simulink model "detectors"  (R2019b)
settings: Solver=VariableStepAuto  StartTime=0.0  StopTime=10.0  RelTol=1e-3
values from neighbouring files (symbols this model uses):
  beta = 0.01    [var.mat]
  c = 2    [var.mat]
  m = 4    [var.mat]
  mu = 0.8    [var.mat]
  omega = 1    [var.mat]
  r = 5    [var.mat]
  s = 1.5    [var.mat]
  steadyVal = 10    [var.mat]
  zeta = 0.5    [var.mat]
libraries: mySTLLib x28
settings Model: Creator=yuxia  LastModifiedBy=yuxia
settings SolverCC: ZeroCrossAlgorithm=Adaptive
settings DebuggingCC: IgnoredZcDiagnostic=none

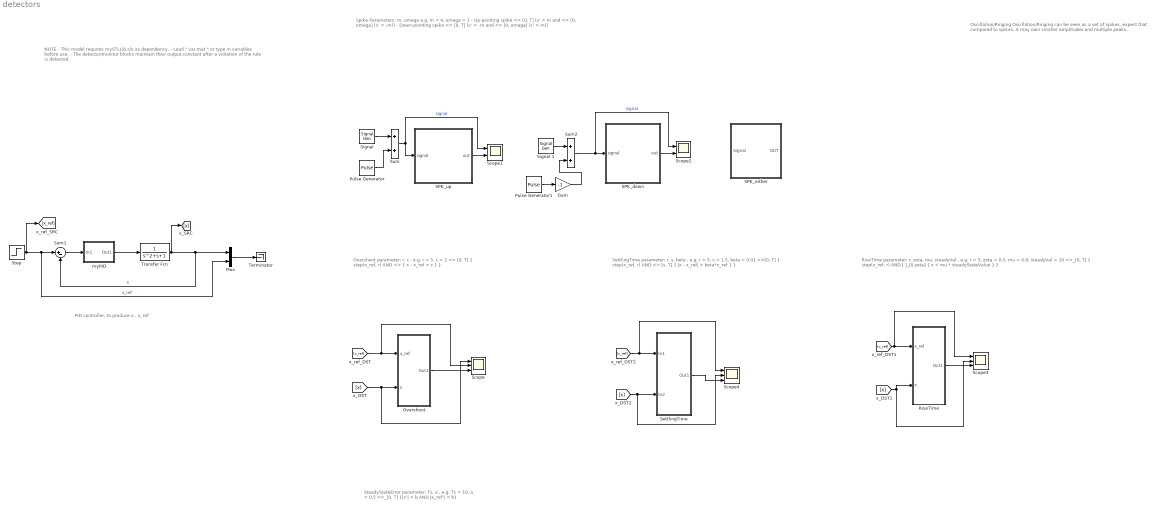
== system detectors ==
  note: PID controller, to produce x , x_ref
  note: Overshoot
      |
      | parameter: r, c , e.g. r = 5, c = 2
      | <> [0, T] { step(x_ref, r) AND <> { x - x_ref > c } }
  note: NOTE
      |
      | - This model requires mySTLLib.slx as dependency.
      |
      | - Load " var.mat " or type in variables before use.
      |
      | - The detector/monitor blocks maintain their output constant after a violation of the rule is detected.
  note: Spike
      |
      | Parameters: m, omega e.g. m = 4, omega = 1
      |
      | - Up-pointing spike
      | <> [0, T] (s' > m and <> [0, omega] (s' < -m))
      |
      | - Down-pointing spike
      | <> [0, T] (s' < -m and <> [0, omega] (s' > m))
  note: Oscillation/Ringing
      |
      | Oscillation/Ringing can be seen as a set of spikes, expect that compared to spikes, it may own smaller amplitudes and multiple peaks.
  note: SettlingTime
      |
      | parameter: r, s, beta , e.g. r = 5, s = 1.5, beta = 0.01
      |
      | <>[0, T] { step(x_ref, r) AND <> [s, T] { |x - x_ref| > beta*x_ref } }
  note: RiseTime
      |
      | parameter: r, zeta, mu, steadyVal , e.g. r = 5, zeta = 0.5, mu = 0.8, steadyVal = 10
      |
      | <>_[0, T] { step(x_ref, r) AND [ ]_[0,zeta] { x < mu * steadyStateValue } }
  note: SteadyStateError
      |
      | parameter: Ts, a , e.g. Ts = 10, a = 0.5
      |
      | <>_[0, T] {|x'| < b AND |x_ref'| < b}
  Gain : Gain  Gain=-1
  Mux : Mux  Inputs=2
  Overshoot : Subsystem
  Pulse Generator : DiscretePulseGenerator  PulseType=Time based  Period=10  PhaseDelay=3.3
  Pulse Generator1 : DiscretePulseGenerator  PulseType=Time based  Period=10  PhaseDelay=3.3
  RiseTime : Subsystem
  SPK_down : Subsystem
  SPK_either : Subsystem
  SPK_up : Subsystem
  Scope : Scope  NumInputPorts=3
  Scope1 : Scope  NumInputPorts=2
  Scope2 : Scope  NumInputPorts=2
  Scope3 : Scope  NumInputPorts=3
  Scope4 : Scope  NumInputPorts=3
  SettlingTime : Subsystem
  "Signal " : SignalGenerator  WaveForm=square  Units=rad/sec
  Signal 1 : SignalGenerator  WaveForm=square  Units=rad/sec
  Step : Step  After=10  SampleTime=0
  Sum : Sum
  Sum1 : Sum  Inputs=|+-
  Sum2 : Sum
  Terminator : Terminator
  Transfer Fcn : TransferFcn  Denominator=[1 1 1]
  myPID : Subsystem
  wires:
  SPK_up/1("out ") -> Scope1/2
  "Signal "/1 -> Sum/1
  Sum/1 -> Scope1/1, SPK_up/1(signal)  "signal"
  [x_ref] -> Scope/2, Overshoot/1(x_ref)
  [x] -> Scope/1, Overshoot/2(x)
  Overshoot/1(Out1) -> Scope/3
  Transfer Fcn/1 -> Mux/1, Sum1/2, [x]  "x"
  myPID/1(Out1) -> Transfer Fcn/1
  Step/1 -> Mux/2, Sum1/1, [x_ref]  "x_ref"
  Sum1/1 -> myPID/1(In1)
  Mux/1 -> Terminator/1
  Sum2/1 -> Scope2/1, SPK_down/1(signal)  "signal"
  SPK_down/1("out ") -> Scope2/2
  Pulse Generator1/1 -> Gain/1
  Signal 1/1 -> Sum2/1
  [x_ref] -> Scope4/1, SettlingTime/1(In1)
  [x] -> SettlingTime/2(In2), Scope4/2
  SettlingTime/1(Out1) -> Scope4/3
  Gain/1 -> Sum2/2
  Pulse Generator/1 -> Sum/2
  [x_ref] -> Scope3/1, RiseTime/1("x_ref ")
  [x] -> Scope3/2, RiseTime/2(x)
  RiseTime/1(Out1) -> Scope3/3

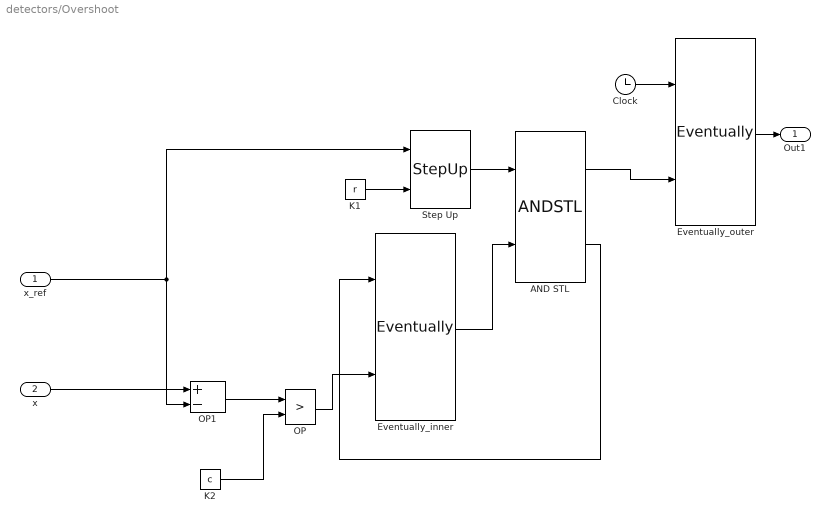
== system detectors/Overshoot ==
  x_ref : Inport
  x : Inport  Port=2
  AND STL : mySTLLib/ANDSTL  SystemSampleTime=-1  Latency=0  AutoFrameSizeCalculation=off
      settings: SourceProductName=My STL Library
  Clock : Clock
  Eventually_inner : mySTLLib/Eventually  SystemSampleTime=-1  Latency=0  AutoFrameSizeCalculation=off
      settings: SourceProductName=My STL Library
  Eventually_outer : mySTLLib/Eventually  SystemSampleTime=-1  Latency=0  AutoFrameSizeCalculation=off
      settings: SourceProductName=My STL Library
  "K1 " : Constant  Value=r
  K2 : Constant  Value=c
  OP : RelationalOperator  Operator=>  OutDataTypeStr=boolean  RndMeth=Simplest
  OP1 : Sum  Inputs=+-
  Step Up : mySTLLib/StepUp  SystemSampleTime=-1  Latency=0  AutoFrameSizeCalculation=off
      settings: SourceProductName=My STL Library
  Out1 : Outport
  wires:
  "K1 "/1 -> Step Up/2
  AND STL/2 -> Eventually_inner/1
  x/1 -> OP1/1
  OP1/1 -> OP/1
  Eventually_outer/1 -> Out1/1
  x_ref/1 -> Step Up/1, OP1/2
  Step Up/1 -> AND STL/1
  OP/1 -> Eventually_inner/2
  AND STL/1 -> Eventually_outer/2
  K2/1 -> OP/2
  Clock/1 -> Eventually_outer/1
  Eventually_inner/1 -> AND STL/2

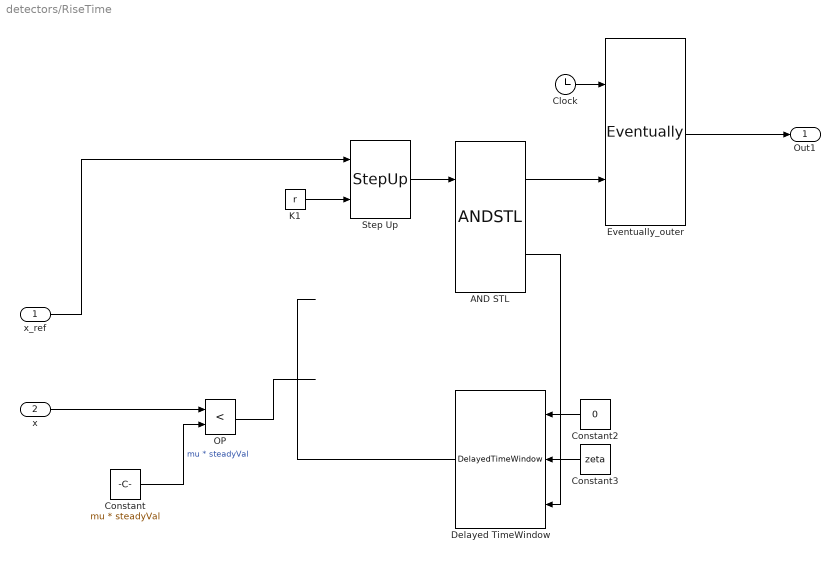
== system detectors/RiseTime ==
  "x_ref " : Inport
  x : Inport  Port=2
  AND STL : mySTLLib/ANDSTL  SystemSampleTime=-1  Latency=0  AutoFrameSizeCalculation=off
      settings: SourceProductName=My STL Library
  Clock : Clock
  Constant : Constant  Value=mu * steadyVal
  Constant2 : Constant  Value=0
  Constant3 : Constant  Value=zeta
  Delayed TimeWindow : mySTLLib/DelayedTimeWindow  SystemSampleTime=-1  Latency=0  AutoFrameSizeCalculation=off
      settings: SourceProductName=My STL Library
  Eventually_outer : mySTLLib/Eventually  SystemSampleTime=-1  Latency=0  AutoFrameSizeCalculation=off
      settings: SourceProductName=My STL Library
  "K1 " : Constant  Value=r
  OP : RelationalOperator  Operator=<  OutDataTypeStr=boolean  RndMeth=Simplest
  Step Up : mySTLLib/StepUp  SystemSampleTime=-1  Latency=0  AutoFrameSizeCalculation=off
      settings: SourceProductName=My STL Library
  Out1 : Outport
  wires:
  "K1 "/1 -> Step Up/2
  Constant/1 -> OP/2  "mu * steadyVal"
  AND STL/1 -> Eventually_outer/2
  Eventually_outer/1 -> Out1/1
  "x_ref "/1 -> Step Up/1
  ? -> AND STL/2
  Clock/1 -> Eventually_outer/1
  Step Up/1 -> AND STL/1
  Constant2/1 -> Delayed TimeWindow/1
  Constant3/1 -> Delayed TimeWindow/2
  AND STL/2 -> Delayed TimeWindow/3
  x/1 -> OP/1
  OP/1 -> ?
  Delayed TimeWindow/1 -> ?

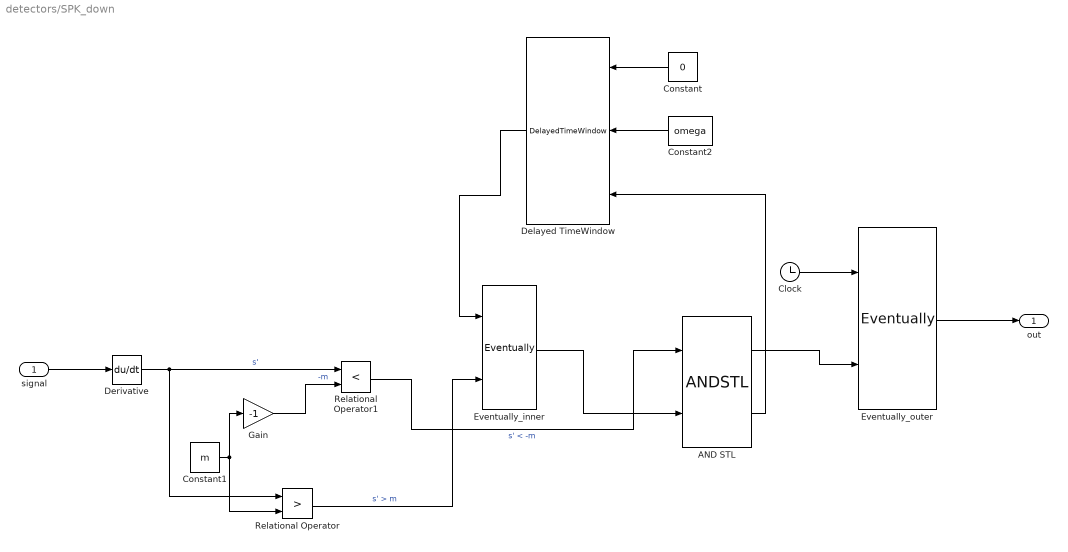
== system detectors/SPK_down ==
  signal : Inport
  AND STL : mySTLLib/ANDSTL  SystemSampleTime=-1  Latency=0  AutoFrameSizeCalculation=off
      settings: SourceProductName=My STL Library
  Clock : Clock
  Constant : Constant  Value=0
  Constant1 : Constant  Value=m
  Constant2 : Constant  Value=omega
  Delayed TimeWindow : mySTLLib/DelayedTimeWindow  SystemSampleTime=-1  Latency=0  AutoFrameSizeCalculation=off
      settings: SourceProductName=My STL Library
  Derivative : Derivative
  Eventually_inner : mySTLLib/Eventually  SystemSampleTime=-1  Latency=0  AutoFrameSizeCalculation=off
      settings: SourceProductName=My STL Library
  Eventually_outer : mySTLLib/Eventually  SystemSampleTime=-1  Latency=0  AutoFrameSizeCalculation=off
      settings: SourceProductName=My STL Library
  Gain : Gain  Gain=-1
  Relational Operator : RelationalOperator  Operator=>  OutDataTypeStr=boolean  RndMeth=Simplest
  Relational Operator1 : RelationalOperator  Operator=<  OutDataTypeStr=boolean  RndMeth=Simplest
  "out " : Outport
  wires:
  Clock/1 -> Eventually_outer/1
  Constant2/1 -> Delayed TimeWindow/2
  Constant1/1 -> Gain/1, Relational Operator/2
  signal/1 -> Derivative/1
  AND STL/2 -> Delayed TimeWindow/3
  Delayed TimeWindow/1 -> Eventually_inner/1
  Eventually_outer/1 -> "out "/1
  Derivative/1 -> Relational Operator1/1, Relational Operator/1  "s'"
  Relational Operator/1 -> Eventually_inner/2  "s' > m"
  Eventually_inner/1 -> AND STL/2
  Constant/1 -> Delayed TimeWindow/1
  Gain/1 -> Relational Operator1/2  "-m"
  AND STL/1 -> Eventually_outer/2
  Relational Operator1/1 -> AND STL/1  "s' < -m"

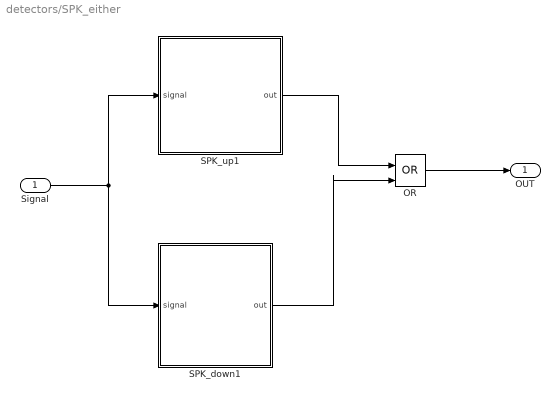
== system detectors/SPK_either ==
  Signal : Inport
  OR : Logic  Operator=OR  IconShape=distinctive  AllPortsSameDT=off  OutDataTypeStr=boolean
  SPK_down1 : Subsystem
  SPK_up1 : Subsystem
  OUT : Outport
  wires:
  Signal/1 -> SPK_up1/1(signal), SPK_down1/1(signal)
  OR/1 -> OUT/1
  SPK_up1/1("out ") -> OR/1
  SPK_down1/1("out ") -> OR/2

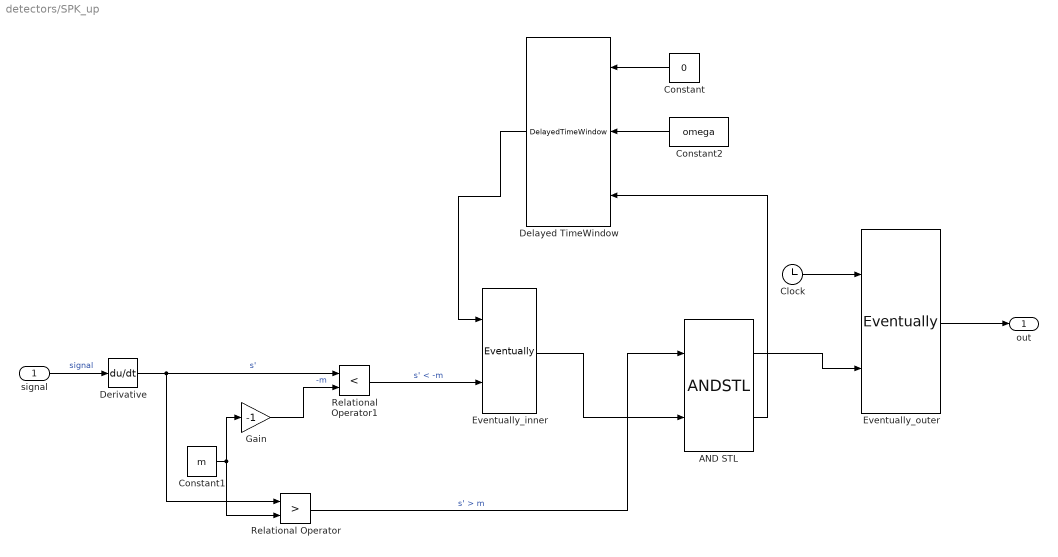
== system detectors/SPK_up ==
  signal : Inport
  AND STL : mySTLLib/ANDSTL  SystemSampleTime=-1  Latency=0  AutoFrameSizeCalculation=off
      settings: SourceProductName=My STL Library
  Clock : Clock
  Constant : Constant  Value=0
  Constant1 : Constant  Value=m
  Constant2 : Constant  Value=omega
  Delayed TimeWindow : mySTLLib/DelayedTimeWindow  SystemSampleTime=-1  Latency=0  AutoFrameSizeCalculation=off
      settings: SourceProductName=My STL Library
  Derivative : Derivative
  Eventually_inner : mySTLLib/Eventually  SystemSampleTime=-1  Latency=0  AutoFrameSizeCalculation=off
      settings: SourceProductName=My STL Library
  Eventually_outer : mySTLLib/Eventually  SystemSampleTime=-1  Latency=0  AutoFrameSizeCalculation=off
      settings: SourceProductName=My STL Library
  Gain : Gain  Gain=-1
  Relational Operator : RelationalOperator  Operator=>  OutDataTypeStr=boolean  RndMeth=Simplest
  Relational Operator1 : RelationalOperator  Operator=<  OutDataTypeStr=boolean  RndMeth=Simplest
  "out " : Outport
  wires:
  signal/1 -> Derivative/1  "signal"
  Eventually_outer/1 -> "out "/1
  Clock/1 -> Eventually_outer/1
  AND STL/1 -> Eventually_outer/2
  Gain/1 -> Relational Operator1/2  "-m"
  Derivative/1 -> Relational Operator1/1, Relational Operator/1  "s'"
  Relational Operator/1 -> AND STL/1  "s' > m"
  Constant1/1 -> Gain/1, Relational Operator/2
  Relational Operator1/1 -> Eventually_inner/2  "s' < -m"
  Eventually_inner/1 -> AND STL/2
  Delayed TimeWindow/1 -> Eventually_inner/1
  AND STL/2 -> Delayed TimeWindow/3
  Constant/1 -> Delayed TimeWindow/1
  Constant2/1 -> Delayed TimeWindow/2

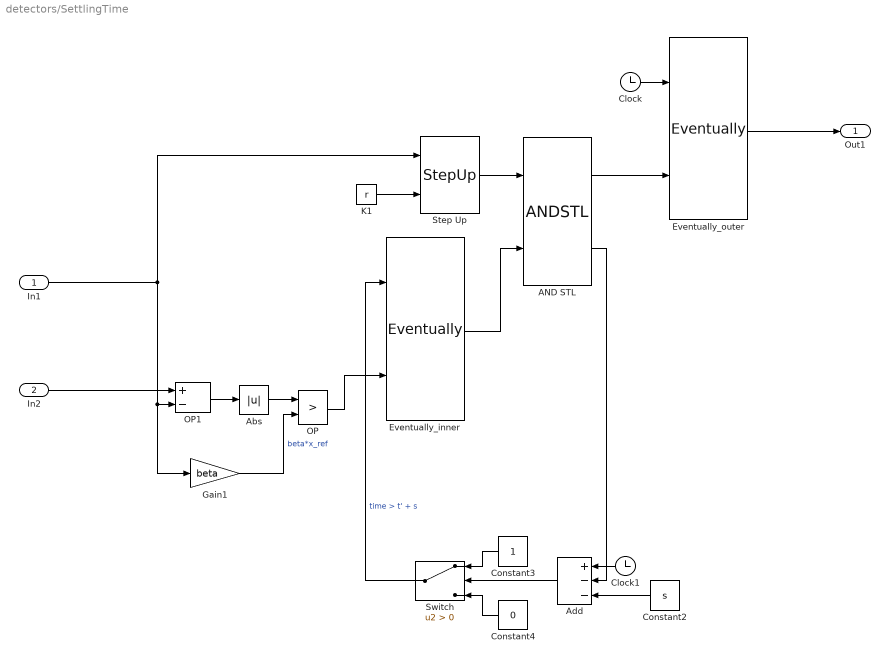
== system detectors/SettlingTime ==
  In1 : Inport
  In2 : Inport  Port=2
  AND STL : mySTLLib/ANDSTL  SystemSampleTime=-1  Latency=0  AutoFrameSizeCalculation=off
      settings: SourceProductName=My STL Library
  Abs : Abs
  Add : Sum  Inputs=+--
  Clock : Clock
  Clock1 : Clock
  Constant2 : Constant  Value=s
  Constant3 : Constant
  Constant4 : Constant  Value=0
  Eventually_inner : mySTLLib/Eventually  SystemSampleTime=-1  Latency=0  AutoFrameSizeCalculation=off
      settings: SourceProductName=My STL Library
  Eventually_outer : mySTLLib/Eventually  SystemSampleTime=-1  Latency=0  AutoFrameSizeCalculation=off
      settings: SourceProductName=My STL Library
  Gain1 : Gain  Gain=beta
  "K1 " : Constant  Value=r
  OP : RelationalOperator  Operator=>  OutDataTypeStr=boolean  RndMeth=Simplest
  OP1 : Sum  Inputs=+-
  Step Up : mySTLLib/StepUp  SystemSampleTime=-1  Latency=0  AutoFrameSizeCalculation=off
      settings: SourceProductName=My STL Library
  Switch : Switch  Criteria=u2 > Threshold
  Out1 : Outport
  wires:
  Gain1/1 -> OP/2  "beta*x_ref"
  Abs/1 -> OP/1
  "K1 "/1 -> Step Up/2
  OP/1 -> Eventually_inner/2
  In2/1 -> OP1/1
  Eventually_outer/1 -> Out1/1
  In1/1 -> Gain1/1, OP1/2, Step Up/1
  Step Up/1 -> AND STL/1
  AND STL/1 -> Eventually_outer/2
  Clock/1 -> Eventually_outer/1
  Eventually_inner/1 -> AND STL/2
  OP1/1 -> Abs/1
  AND STL/2 -> Add/2
  Clock1/1 -> Add/1
  Constant2/1 -> Add/3
  Add/1 -> Switch/2
  Constant3/1 -> Switch/1
  Constant4/1 -> Switch/3
  Switch/1 -> Eventually_inner/1  "time > t' + s"

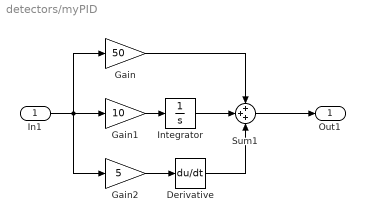
== system detectors/myPID ==
  In1 : Inport
  Derivative : Derivative
  Gain : Gain  Gain=50
  Gain1 : Gain  Gain=10
  Gain2 : Gain  Gain=5
  Integrator : Integrator
  Sum1 : Sum  Inputs=+++
  Out1 : Outport
  wires:
  Derivative/1 -> Sum1/3
  Integrator/1 -> Sum1/2
  Gain/1 -> Sum1/1
  In1/1 -> Gain2/1, Gain/1, Gain1/1
  Sum1/1 -> Out1/1
  Gain1/1 -> Integrator/1
  Gain2/1 -> Derivative/1

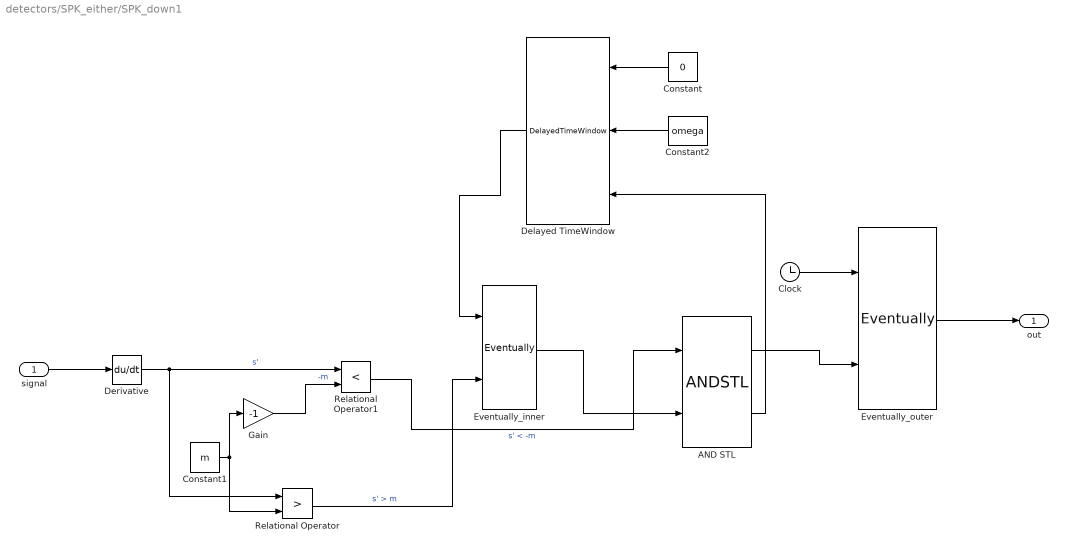
== system detectors/SPK_either/SPK_down1 ==
  signal : Inport
  AND STL : mySTLLib/ANDSTL  SystemSampleTime=-1  Latency=0  AutoFrameSizeCalculation=off
      settings: SourceProductName=My STL Library
  Clock : Clock
  Constant : Constant  Value=0
  Constant1 : Constant  Value=m
  Constant2 : Constant  Value=omega
  Delayed TimeWindow : mySTLLib/DelayedTimeWindow  SystemSampleTime=-1  Latency=0  AutoFrameSizeCalculation=off
      settings: SourceProductName=My STL Library
  Derivative : Derivative
  Eventually_inner : mySTLLib/Eventually  SystemSampleTime=-1  Latency=0  AutoFrameSizeCalculation=off
      settings: SourceProductName=My STL Library
  Eventually_outer : mySTLLib/Eventually  SystemSampleTime=-1  Latency=0  AutoFrameSizeCalculation=off
      settings: SourceProductName=My STL Library
  Gain : Gain  Gain=-1
  Relational Operator : RelationalOperator  Operator=>  OutDataTypeStr=boolean  RndMeth=Simplest
  Relational Operator1 : RelationalOperator  Operator=<  OutDataTypeStr=boolean  RndMeth=Simplest
  "out " : Outport
  wires:
  Clock/1 -> Eventually_outer/1
  Constant2/1 -> Delayed TimeWindow/2
  Constant1/1 -> Gain/1, Relational Operator/2
  signal/1 -> Derivative/1
  AND STL/2 -> Delayed TimeWindow/3
  Delayed TimeWindow/1 -> Eventually_inner/1
  Eventually_outer/1 -> "out "/1
  Derivative/1 -> Relational Operator1/1, Relational Operator/1  "s'"
  Relational Operator/1 -> Eventually_inner/2  "s' > m"
  Eventually_inner/1 -> AND STL/2
  Constant/1 -> Delayed TimeWindow/1
  Gain/1 -> Relational Operator1/2  "-m"
  AND STL/1 -> Eventually_outer/2
  Relational Operator1/1 -> AND STL/1  "s' < -m"

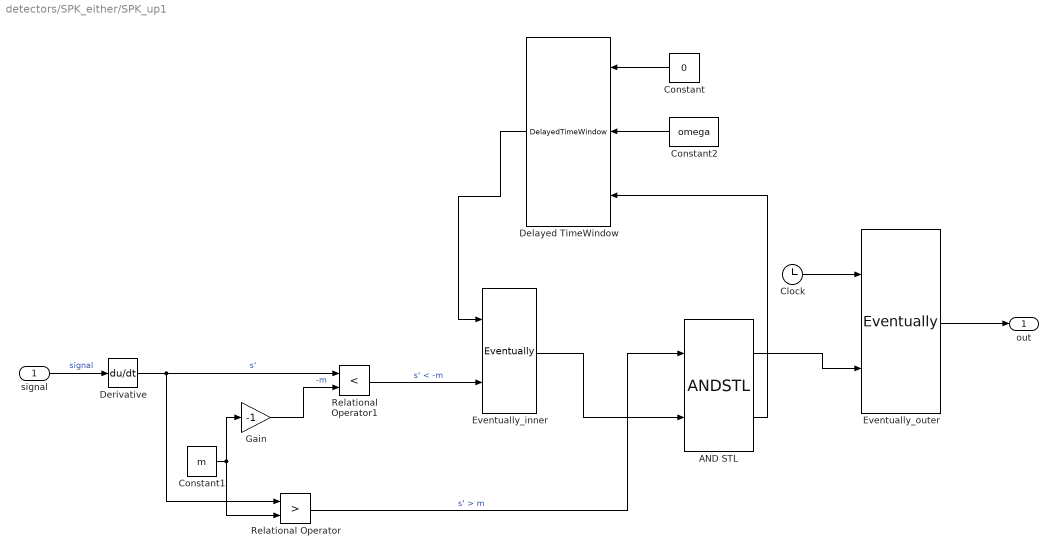
== system detectors/SPK_either/SPK_up1 ==
  signal : Inport
  AND STL : mySTLLib/ANDSTL  SystemSampleTime=-1  Latency=0  AutoFrameSizeCalculation=off
      settings: SourceProductName=My STL Library
  Clock : Clock
  Constant : Constant  Value=0
  Constant1 : Constant  Value=m
  Constant2 : Constant  Value=omega
  Delayed TimeWindow : mySTLLib/DelayedTimeWindow  SystemSampleTime=-1  Latency=0  AutoFrameSizeCalculation=off
      settings: SourceProductName=My STL Library
  Derivative : Derivative
  Eventually_inner : mySTLLib/Eventually  SystemSampleTime=-1  Latency=0  AutoFrameSizeCalculation=off
      settings: SourceProductName=My STL Library
  Eventually_outer : mySTLLib/Eventually  SystemSampleTime=-1  Latency=0  AutoFrameSizeCalculation=off
      settings: SourceProductName=My STL Library
  Gain : Gain  Gain=-1
  Relational Operator : RelationalOperator  Operator=>  OutDataTypeStr=boolean  RndMeth=Simplest
  Relational Operator1 : RelationalOperator  Operator=<  OutDataTypeStr=boolean  RndMeth=Simplest
  "out " : Outport
  wires:
  signal/1 -> Derivative/1  "signal"
  Eventually_outer/1 -> "out "/1
  Clock/1 -> Eventually_outer/1
  AND STL/1 -> Eventually_outer/2
  Gain/1 -> Relational Operator1/2  "-m"
  Derivative/1 -> Relational Operator1/1, Relational Operator/1  "s'"
  Relational Operator/1 -> AND STL/1  "s' > m"
  Constant1/1 -> Gain/1, Relational Operator/2
  Relational Operator1/1 -> Eventually_inner/2  "s' < -m"
  Eventually_inner/1 -> AND STL/2
  Delayed TimeWindow/1 -> Eventually_inner/1
  AND STL/2 -> Delayed TimeWindow/3
  Constant/1 -> Delayed TimeWindow/1
  Constant2/1 -> Delayed TimeWindow/2
